simulink model "basic_control_structure"  (Simulink 6.3)
settings: Solver=ode45  StartTime=0.0  StopTime=6174  RelTol=1e-3
undefined symbols (not defined in the file): A_ang_c, B_ang_c, C_ang_c, D_ang_c
libraries: components_lib x4, simulink x1
settings Model: Creator=krage  LastModifiedBy=mnkr02  ExtModeAutoUpdateStatusClock=off  StrictBusMsg=None
settings DebuggingCC: CheckSSInitialOutputMsg=off

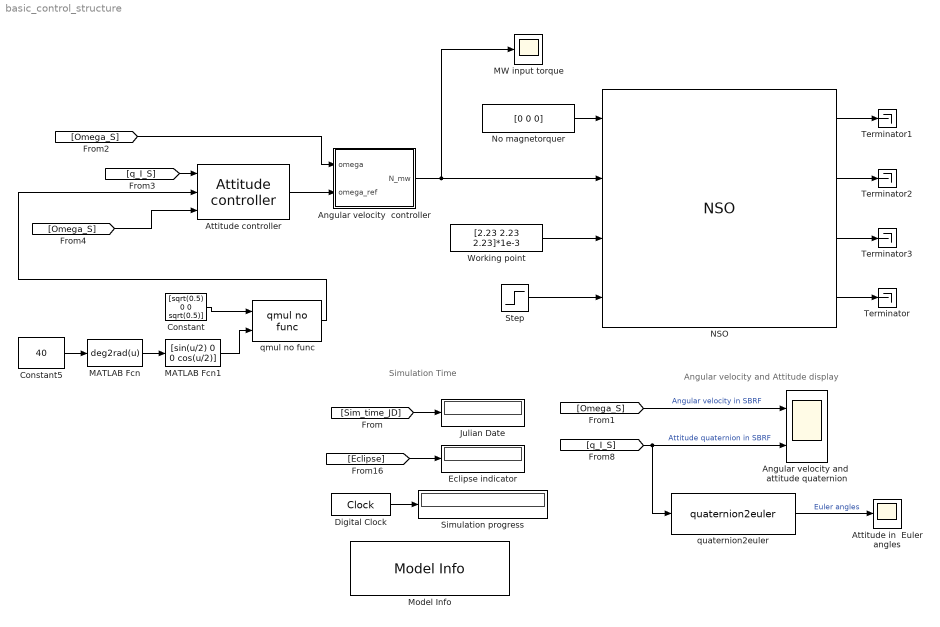
== system basic_control_structure ==
  note: Simulation Time
  note: Angular velocity and Attitude display
  Angular velocity  controller : Subsystem  mask(Angular Velocity Controller){ang_file_name='basic_ang_control.m'}
      mask prompts: ang_file_name "Angular rate controller design file name (remember gnyfs :-))"
      mask help:
      | The controller in this block is to be constructed using a state space system. The
      | reference is subtracted from the measurement (positive feedback and SS-reference) and passed through the SS-system. Thus if the controller is merely a gain matrix only the D-matrix has to contain the controller and the remaining be zero-matrices. The controller design files are kept in the "design" directory and the definition of the controller system matrices is the final task in each controller design file.
      | The different matrices for the state space system are named:
      | A_ang_c
      | B_ang_c
      | C_ang_c
      | D_ang_c
      mask init:
      | run(strcat('design/',ang_file_name))
  Angular velocity and  attitude quaternion : Scope  NumInputPorts=2
      settings: YMin=-250~-1  YMax=1250~1
  Attitude controller : components_lib/ACS/Controllers/Attitude controller  att_file_name='attitude_control_lqr.m'
  Attitude in  Euler angles : Scope
      settings: YMin=-3.5  YMax=3.5
  Constant : Constant  Value=[sqrt(0.5) 0 0 sqrt(0.5)]
  Constant5 : Constant  Value=40
  Digital Clock : DigitalClock
  Eclipse indicator : Display
  Julian Date : Display
  MATLAB Fcn : MATLABFcn  MATLABFcn=deg2rad(u)
  MATLAB Fcn1 : MATLABFcn  MATLABFcn=[sin(u/2) 0 0 cos(u/2)]
  MW input torque : Scope
      settings: YMin=-7e-06  YMax=6e-06  SaveName=ScopeData6
  Model Info : simulink/Model-Wide Utilities/Model Info  InitialBlockCM=None  BlockCM=None  Frame=on  DisplayStringWithTags=|  HorizontalTextAlignment=Left  LeftAlignmentValue=0.02  SourceBlockDiagram=basic_control_structure  TagMaxNumber=20
      | Usefull Julian dates:
      | sun to eclipse : 2452315.560376
      | 32 sec. before : 2452315.56
      | eclipse to sun : 2452315.513363
  NSO : components_lib/NSO  Tag=AAUSAT-II Model  Description=AAUSAT-II Model  r_com_s=[0.05 0.05 0.15]  sat_temp_start=0  r_com_s_deployed=[0.05 0.05 0.125]  mass_sc=3  Dim=[0.1 0.1 0.3]  inertia_c=[25 25 5]/1e3  inertia_d=[42.3 42.3 28.4]/1e3  init_jd=2452315.56  q_s_c=[0 0 0 1]  q_init_s_i=[sqrt(0.5) 0 0 sqrt(0.5)]  w_init_s=[0.1 0.1 0.1]  Cd=2  rho=9.25e-13  enable_sensor_emulation=off  alb_emu_enabled=off  enable_dist=off
  No magnetorquer : Constant  Value=[0 0 0]
  Simulation progress : Display
  Step : Step  Time=0  SampleTime=0
  Terminator{,1..3} (4 alike) : Terminator
  Working point : Constant  Value=[2.23 2.23 2.23]*1e-3
  qmul no func : components_lib/Math utilities/Quaternion operations/qmul no func
  quaternion2euler : components_lib/Math utilities/Quaternion operations/quaternion2euler
  wires:
  [Omega_S] -> Angular velocity and  attitude quaternion/1  "Angular velocity in SBRF"
  [q_I_S] -> quaternion2euler/1, Angular velocity and  attitude quaternion/2  "Attitude quaternion in SBRF"
  quaternion2euler/1 -> Attitude in  Euler angles/1  "Euler angles"
  [Sim_time_JD] -> Julian Date/1
  [Eclipse] -> Eclipse indicator/1
  Digital Clock/1 -> Simulation progress/1
  Step/1 -> NSO/4
  Working point/1 -> NSO/3
  Angular velocity  controller/1(N_mw) -> NSO/2, MW input torque/1
  [Omega_S] -> Angular velocity  controller/1(omega)
  NSO/1 -> Terminator1/1
  NSO/2 -> Terminator2/1
  NSO/3 -> Terminator3/1
  NSO/4 -> Terminator/1
  No magnetorquer/1 -> NSO/1
  qmul no func/1 -> Attitude controller/2
  [q_I_S] -> Attitude controller/1
  Attitude controller/1 -> Angular velocity  controller/2(omega_ref)
  [Omega_S] -> Attitude controller/3
  Constant5/1 -> MATLAB Fcn/1
  MATLAB Fcn/1 -> MATLAB Fcn1/1
  MATLAB Fcn1/1 -> qmul no func/2
  Constant/1 -> qmul no func/1

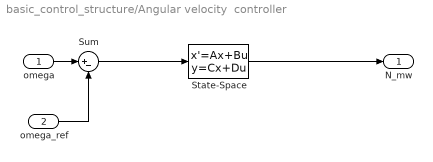
== system basic_control_structure/Angular velocity  controller ==
  omega : Inport
  omega_ref : Inport  Port=2
  State-Space : StateSpace  A=A_ang_c  B=B_ang_c  C=C_ang_c  D=D_ang_c
  Sum : Sum  Inputs=|+-
  N_mw : Outport
  wires:
  Sum/1 -> State-Space/1
  State-Space/1 -> N_mw/1
  omega/1 -> Sum/1
  omega_ref/1 -> Sum/2
